simulink model "CLRC_Panda_SP_A"  (R2023a)
settings: Solver=ode3  StartTime=0.0  StopTime=105  FixedStep=Ts  MaxStep=0.005  RelTol=1e-5
model workspace (MAT data in the model file):
  SL_ROS_VariableLengthArrays_MaxSizes.CommonInfo.ArrayTruncateAction = 'EmitWarning'
  SL_ROS_VariableLengthArrays_MaxSizes.MsgTypeMap = containers.Map
  SL_ROS_VariableLengthArrays_MaxSizes.MsgTypeMap.serialization.keys = {'gazebo_msgs/ApplyJointEffortRequest', 'sensor_msgs/JointState'}
  SL_ROS_VariableLengthArrays_MaxSizes.MsgTypeMap.serialization.values{1}.PropertyName = 'JointName'
  SL_ROS_VariableLengthArrays_MaxSizes.MsgTypeMap.serialization.values{1}.DataType = 'uint8'
  SL_ROS_VariableLengthArrays_MaxSizes.MsgTypeMap.serialization.values{1}.MaxLength = 12
  SL_ROS_VariableLengthArrays_MaxSizes.MsgTypeMap.serialization.values{2}(1).PropertyName = 'Effort'
  SL_ROS_VariableLengthArrays_MaxSizes.MsgTypeMap.serialization.values{2}(1).DataType = 'double'
  SL_ROS_VariableLengthArrays_MaxSizes.MsgTypeMap.serialization.values{2}(1).MaxLength = 128
  SL_ROS_VariableLengthArrays_MaxSizes.MsgTypeMap.serialization.values{2}(2).PropertyName = 'Name'
  SL_ROS_VariableLengthArrays_MaxSizes.MsgTypeMap.serialization.values{2}(2).DataType = 'std_msgs/String'
  SL_ROS_VariableLengthArrays_MaxSizes.MsgTypeMap.serialization.values{2}(2).MaxLength = 16
  SL_ROS_VariableLengthArrays_MaxSizes.MsgTypeMap.serialization.values{2}(3).PropertyName = 'Position'
  SL_ROS_VariableLengthArrays_MaxSizes.MsgTypeMap.serialization.values{2}(3).DataType = 'double'
  SL_ROS_VariableLengthArrays_MaxSizes.MsgTypeMap.serialization.values{2}(3).MaxLength = 7
  SL_ROS_VariableLengthArrays_MaxSizes.MsgTypeMap.serialization.values{2}(4).PropertyName = 'Velocity'
  SL_ROS_VariableLengthArrays_MaxSizes.MsgTypeMap.serialization.values{2}(4).DataType = 'double'
  SL_ROS_VariableLengthArrays_MaxSizes.MsgTypeMap.serialization.values{2}(4).MaxLength = 7
  SL_ROS_VariableLengthArrays_MaxSizes.MsgTypeMap.serialization.uniformity = 0
  SL_ROS_VariableLengthArrays_MaxSizes.MsgTypeMap.serialization.keyType = 'char'
  SL_ROS_VariableLengthArrays_MaxSizes.MsgTypeMap.serialization.valueType = 'any'
values from neighbouring files (symbols this model uses):
  B = 4.44*I    [Panda_run.m]
  D = 0.1075*I    [Panda_run.m]
  eKd = 1*inv(K)*B*2*omega_n-inv(K)*D    [Panda_run.m]
  K = 14000*I    [Panda_run.m]
  Kc = diag([20,20,20,20,8,8,5])*0.5    [Panda_run.m]
  Kp = kpdata    [Kp_Compare.m]    (also in Panda_run.m = kp*I)
  Lambda = 10*eye(7)*0.5    [Panda_run.m]
  par = baseparmes()    [Panda_run.m]
  q0 = traj.qd.Data(:,:,1)    [Panda_run.m]
  SD = 0    [Panda_run.m]
  Ts = 0.0005    [Kp_Compare.m]    (also in Panda_run.m)
  vari = SD^2    (= 0)    [Panda_run.m]
undefined symbols (not defined in the file or in its folder): gravityMatrix
libraries: matrix_library x1
settings Model: Creator=STT  LastModifiedBy=stt
settings OptimizationCC: DefaultParameterBehavior=Inlined  EnhancedBackFolding=on  PassReuseOutputArgsAs=Individual arguments  ZeroExternalMemoryAtStartup=off  ZeroInternalMemoryAtStartup=off  MaxStackSize=64  AccelVerboseBuild=on  OptimizeBlockOrder=speed  DifferentSizesBufferReuse=on  OptimizationCustomize=off  EfficientTunableParamExpr=on
settings DebuggingCC: AlgebraicLoopMsg=error  ArtificialAlgebraicLoopMsg=error  ParameterTunabilityLossMsg=error  UnconnectedInputMsg=warning  UnconnectedOutputMsg=warning  UnconnectedLineMsg=warning
settings HardwareCC: ProdHWDeviceType=AMD->x86-64 (Windows64)
settings ModelReferenceCC: EnableRefExpFcnMdlSchedulingChecks=on
settings SFSimCC: MATLABDynamicMemAlloc=off
settings RTWCC: Description=Embedded Coder  SystemTargetFile=ert.tlc  TemplateMakefile=ert_default_tmf  Toolchain=Catkin  DLArmComputeVersion=19.05
settings CodeAppCC: ForceParamTrailComments=on  IgnoreCustomStorageClasses=off  OperatorAnnotations=on  SimulinkDataObjDesc=on  SFDataObjDesc=on  InsertBlockDesc=on
settings ERTTargetCC: SupportContinuousTime=on  SupportVariableSizeSignals=on  ExtMode=on  ExtModeMexArgs='192.168.175.128' 0 17725  ERTCustomFileTemplate=example_file_process.tlc

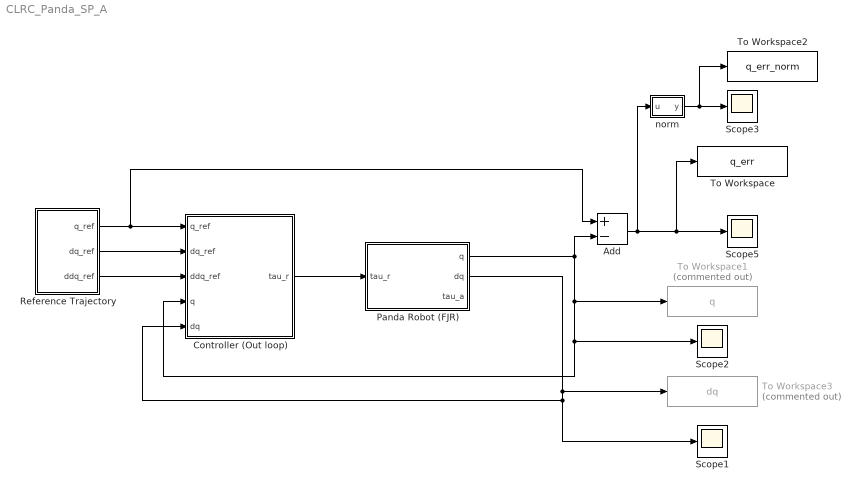
== system CLRC_Panda_SP_A ==
  Add : Sum  Inputs=+-
  Controller (Out loop) : Subsystem
  Panda Robot (FJR) : Subsystem
  Reference Trajectory : Subsystem
  Scope{1..3,5} (4 alike) : Scope
  To Workspace : ToWorkspace  VariableName=q_err  SaveFormat=Timeseries  SampleTime=-1
  To Workspace1 : ToWorkspace  Commented=on  VariableName=q  SaveFormat=Timeseries  SampleTime=-1
  To Workspace2 : ToWorkspace  VariableName=q_err_norm  SaveFormat=Timeseries  SampleTime=-1
  To Workspace3 : ToWorkspace  Commented=on  VariableName=dq  SaveFormat=Timeseries  SampleTime=-1
  norm : MATLAB Function  TreatAsAtomicUnit=on
  wires:
  Reference Trajectory/1(q_ref) -> Add/1, Controller (Out loop)/1(q_ref)
  Reference Trajectory/2(dq_ref) -> Controller (Out loop)/2(dq_ref)
  Reference Trajectory/3(ddq_ref) -> Controller (Out loop)/3(ddq_ref)
  Add/1 -> norm/1(u), Scope5/1, To Workspace/1
  Panda Robot (FJR)/2(dq) -> Scope1/1, Controller (Out loop)/5(dq), To Workspace3/1
  Panda Robot (FJR)/1(q) -> Add/2, Controller (Out loop)/4(q), Scope2/1, To Workspace1/1
  norm/1(y) -> To Workspace2/1, Scope3/1
  Controller (Out loop)/1(tau_r) -> Panda Robot (FJR)/1(tau_r)

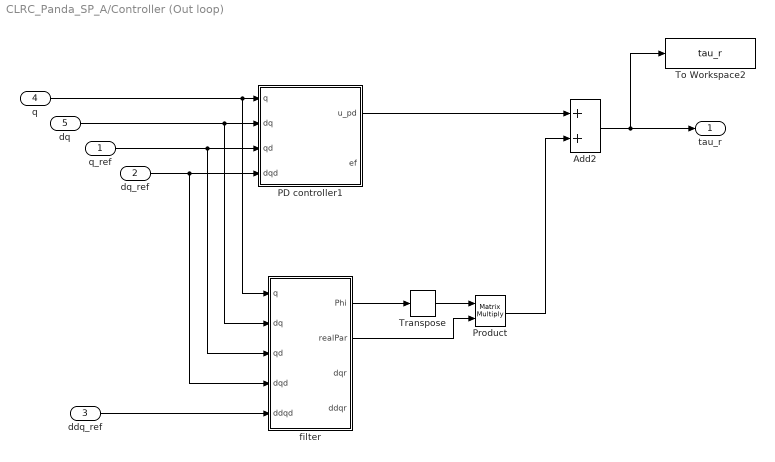
== system CLRC_Panda_SP_A/Controller (Out loop) ==
  q_ref : Inport
  dq_ref : Inport  Port=2
  ddq_ref : Inport  Port=3
  q : Inport  Port=4
  dq : Inport  Port=5
  Add2 : Sum
  PD controller1 : Subsystem
  Product : Product  Multiplication=Matrix(*)
  To Workspace2 : ToWorkspace  VariableName=tau_r  SaveFormat=Timeseries  SampleTime=-1
  Transpose : matrix_library/Transpose
  filter : Subsystem
  tau_r : Outport
  wires:
  q/1 -> PD controller1/1(q), filter/1(q)
  q_ref/1 -> PD controller1/3(qd), filter/3(qd)
  dq_ref/1 -> PD controller1/4(dqd), filter/4(dqd)
  dq/1 -> PD controller1/2(dq), filter/2(dq)
  PD controller1/1(u_pd) -> Add2/1
  Transpose/1 -> Product/1
  Product/1 -> Add2/2
  filter/1(Phi) -> Transpose/1
  filter/2(realPar) -> Product/2
  ddq_ref/1 -> filter/5(ddqd)
  Add2/1 -> tau_r/1, To Workspace2/1

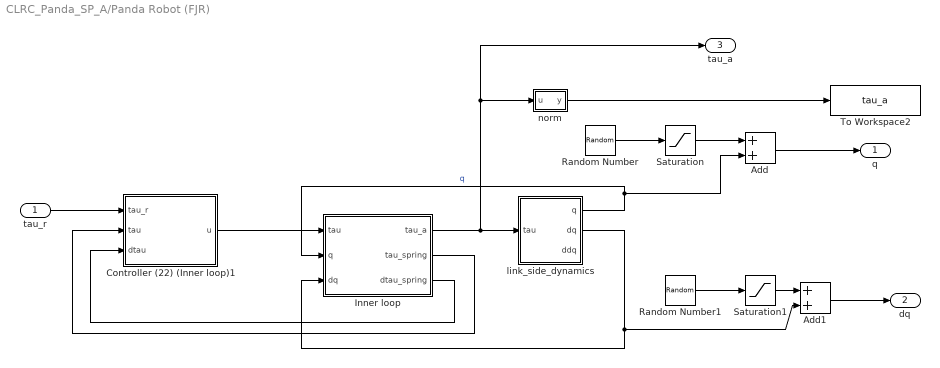
== system CLRC_Panda_SP_A/Panda Robot (FJR) ==
  tau_r : Inport
  Add : Sum
  Add1 : Sum
  Controller (22) (Inner loop)1 : Subsystem
  Inner loop : Subsystem
  Random Number : RandomNumber  Variance=vari  SampleTime=Ts
  Random Number1 : RandomNumber  Variance=vari  SampleTime=Ts
  Saturation : Saturate  UpperLimit=3*SD  LowerLimit=-3*SD
  Saturation1 : Saturate  UpperLimit=3*SD  LowerLimit=-3*SD
  To Workspace2 : ToWorkspace  VariableName=tau_a  SaveFormat=Timeseries  SampleTime=-1
  link_side_dynamics : Subsystem
  norm : MATLAB Function  TreatAsAtomicUnit=on
  q : Outport
  dq : Outport  Port=2
  tau_a : Outport  Port=3
  wires:
  link_side_dynamics/1(q) -> Add/2, Inner loop/2(q)  "q"
  Inner loop/2(tau_spring) -> Controller (22) (Inner loop)1/2(tau)
  Inner loop/3(dtau_spring) -> Controller (22) (Inner loop)1/3(dtau)
  link_side_dynamics/2(dq) -> Inner loop/3(dq), Add1/2
  Controller (22) (Inner loop)1/1(u) -> Inner loop/1(tau)
  norm/1(y) -> To Workspace2/1
  Inner loop/1(tau_a) -> tau_a/1, norm/1(u), link_side_dynamics/1(tau)
  tau_r/1 -> Controller (22) (Inner loop)1/1(tau_r)
  Random Number1/1 -> Saturation1/1
  Saturation/1 -> Add/1
  Random Number/1 -> Saturation/1
  Add/1 -> q/1
  Saturation1/1 -> Add1/1
  Add1/1 -> dq/1

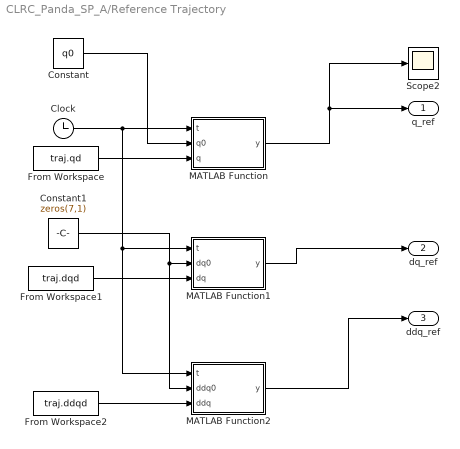
== system CLRC_Panda_SP_A/Reference Trajectory ==
  Clock : Clock
  Constant : Constant  Value=q0
  Constant1 : Constant  Value=zeros(7,1)
  From Workspace : FromWorkspace  VariableName=traj.qd
  From Workspace1 : FromWorkspace  VariableName=traj.dqd
  From Workspace2 : FromWorkspace  VariableName=traj.ddqd
  MATLAB Function : MATLAB Function  TreatAsAtomicUnit=on
  MATLAB Function1 : MATLAB Function  TreatAsAtomicUnit=on
  MATLAB Function2 : MATLAB Function  TreatAsAtomicUnit=on
  Scope2 : Scope
  q_ref : Outport
  dq_ref : Outport  Port=2
  ddq_ref : Outport  Port=3
  wires:
  MATLAB Function/1(y) -> Scope2/1, q_ref/1
  MATLAB Function1/1(y) -> dq_ref/1
  MATLAB Function2/1(y) -> ddq_ref/1
  Clock/1 -> MATLAB Function2/1(t), MATLAB Function1/1(t), MATLAB Function/1(t)
  From Workspace/1 -> MATLAB Function/3(q)
  Constant/1 -> MATLAB Function/2(q0)
  From Workspace1/1 -> MATLAB Function1/3(dq)
  From Workspace2/1 -> MATLAB Function2/3(ddq)
  Constant1/1 -> MATLAB Function2/2(ddq0), MATLAB Function1/2(dq0)

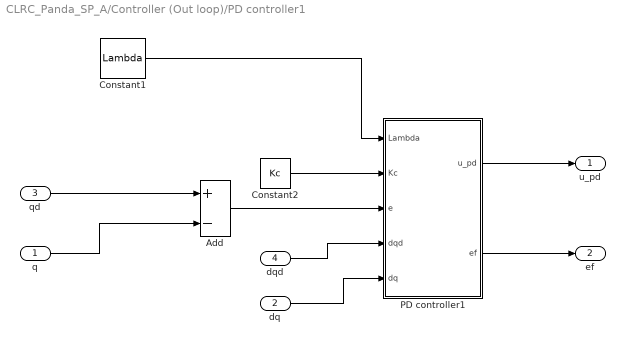
== system CLRC_Panda_SP_A/Controller (Out loop)/PD controller1 ==
  q : Inport
  dq : Inport  Port=2
  qd : Inport  Port=3
  dqd : Inport  Port=4
  Add : Sum  Inputs=+-
  Constant1 : Constant  Value=Lambda
  Constant2 : Constant  Value=Kc
  PD controller1 : MATLAB Function  TreatAsAtomicUnit=on
  u_pd : Outport
  ef : Outport  Port=2
  wires:
  PD controller1/1(u_pd) -> u_pd/1
  Add/1 -> PD controller1/3(e)
  Constant1/1 -> PD controller1/1(Lambda)
  Constant2/1 -> PD controller1/2(Kc)
  PD controller1/2(ef) -> ef/1
  q/1 -> Add/2
  qd/1 -> Add/1
  dq/1 -> PD controller1/5(dq)
  dqd/1 -> PD controller1/4(dqd)

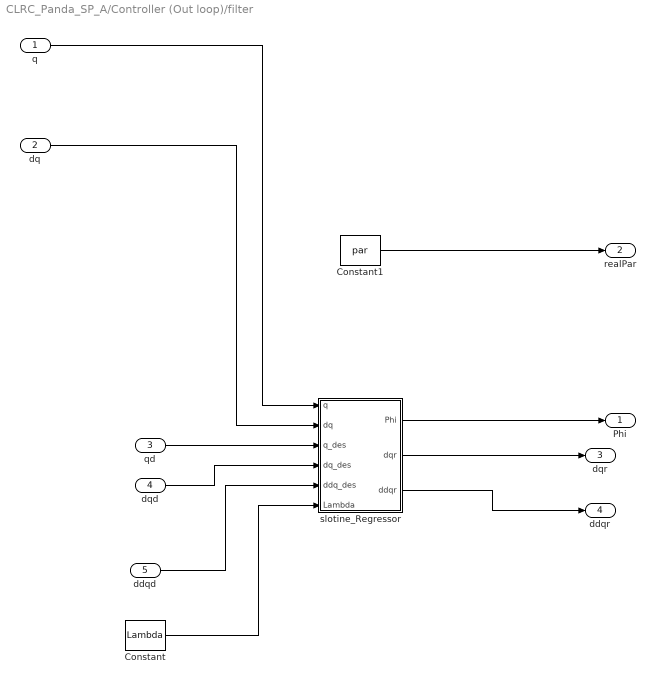
== system CLRC_Panda_SP_A/Controller (Out loop)/filter ==
  q : Inport
  dq : Inport  Port=2
  qd : Inport  Port=3
  dqd : Inport  Port=4
  ddqd : Inport  Port=5
  Constant : Constant  Value=Lambda
  Constant1 : Constant  Value=par
  slotine_Regressor : MATLAB Function  TreatAsAtomicUnit=on
  Phi : Outport
  realPar : Outport  Port=2
  dqr : Outport  Port=3
  ddqr : Outport  Port=4
  wires:
  qd/1 -> slotine_Regressor/3(q_des)
  dqd/1 -> slotine_Regressor/4(dq_des)
  ddqd/1 -> slotine_Regressor/5(ddq_des)
  Constant/1 -> slotine_Regressor/6(Lambda)
  q/1 -> slotine_Regressor/1(q)
  dq/1 -> slotine_Regressor/2(dq)
  Constant1/1 -> realPar/1
  slotine_Regressor/1(Phi) -> Phi/1
  slotine_Regressor/2(dqr) -> dqr/1
  slotine_Regressor/3(ddqr) -> ddqr/1

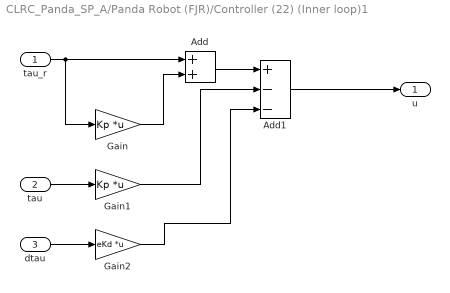
== system CLRC_Panda_SP_A/Panda Robot (FJR)/Controller (22) (Inner loop)1 ==
  tau_r : Inport
  tau : Inport  Port=2
  dtau : Inport  Port=3
  Add : Sum
  Add1 : Sum  Inputs=+--
  Gain : Gain  Gain=Kp  Multiplication=Matrix(K*u)
  Gain1 : Gain  Gain=Kp  Multiplication=Matrix(K*u)
  Gain2 : Gain  Gain=eKd  Multiplication=Matrix(K*u)
  u : Outport
  wires:
  tau/1 -> Gain1/1
  Add/1 -> Add1/1
  Add1/1 -> u/1
  dtau/1 -> Gain2/1
  Gain1/1 -> Add1/2
  tau_r/1 -> Add/1, Gain/1
  Gain/1 -> Add/2
  Gain2/1 -> Add1/3

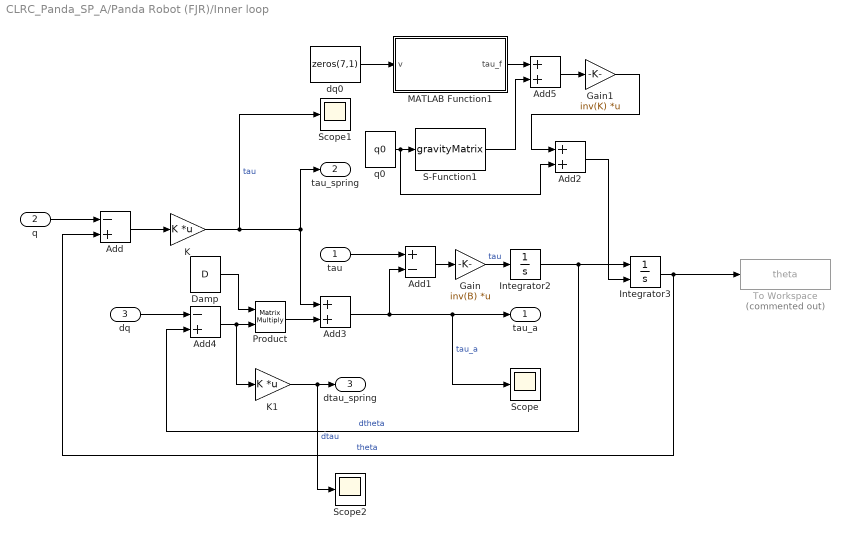
== system CLRC_Panda_SP_A/Panda Robot (FJR)/Inner loop ==
  tau : Inport
  q : Inport  Port=2
  dq : Inport  Port=3
  Add : Sum  Inputs=-+
  Add1 : Sum  Inputs=+-
  Add2 : Sum
  Add3 : Sum
  Add4 : Sum  Inputs=-+
  Add5 : Sum
  Damp : Constant  Value=D
  Gain : Gain  Gain=inv(B)  Multiplication=Matrix(K*u)
  Gain1 : Gain  Gain=inv(K)  Multiplication=Matrix(K*u)
  Integrator2 : Integrator
  Integrator3 : Integrator  InitialConditionSource=external  InitialCondition=q0+K\gravityMatrix(q0)
  K : Gain  Gain=K  Multiplication=Matrix(K*u)
  K1 : Gain  Gain=K  Multiplication=Matrix(K*u)
  MATLAB Function1 : MATLAB Function  TreatAsAtomicUnit=on
  Product : Product  Multiplication=Matrix(*)
  S-Function1 : S-Function  FunctionName=gravityMatrix  SFunctionDeploymentMode=off  EnableBusSupport=off
  Scope : Scope
  Scope1 : Scope
  Scope2 : Scope
  To Workspace : ToWorkspace  Commented=on  VariableName=theta  SaveFormat=Timeseries  SampleTime=-1
  dq0 : Constant  Value=zeros(7,1)
  q0 : Constant  Value=q0
  tau_a : Outport
  tau_spring : Outport  Port=2
  dtau_spring : Outport  Port=3
  wires:
  q/1 -> Add/1
  Add/1 -> K/1
  K/1 -> Scope1/1, tau_spring/1, Add3/1  "tau"
  Product/1 -> Add3/2
  Add1/1 -> Gain/1
  Integrator2/1 -> Integrator3/1, Add4/2  "dtheta"
  Integrator3/1 -> Add/2, To Workspace/1  "theta"
  Add3/1 -> Scope/1, tau_a/1, Add1/2  "tau_a"
  dq/1 -> Add4/1
  Add4/1 -> K1/1, Product/2
  Damp/1 -> Product/1
  K1/1 -> Scope2/1, dtau_spring/1  "dtau"
  tau/1 -> Add1/1
  q0/1 -> Add2/2, S-Function1/1
  Gain1/1 -> Add2/1
  Add2/1 -> Integrator3/2
  dq0/1 -> MATLAB Function1/1(v)
  MATLAB Function1/1(tau_f) -> Add5/1
  Add5/1 -> Gain1/1
  S-Function1/1 -> Add5/2
  Gain/1 -> Integrator2/1  "tau"

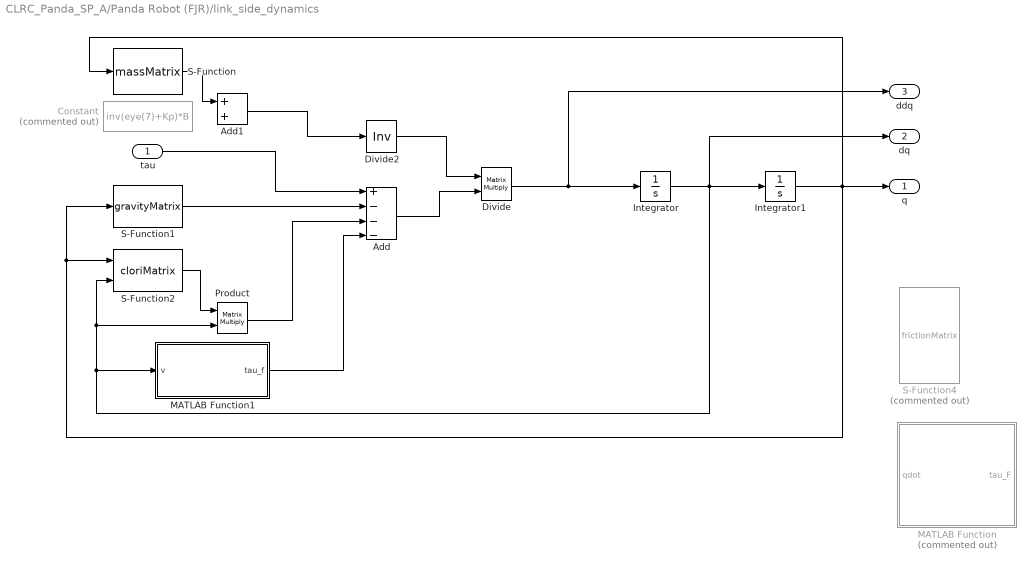
== system CLRC_Panda_SP_A/Panda Robot (FJR)/link_side_dynamics ==
  tau : Inport
  Add : Sum  Inputs=+---
  Add1 : Sum
  Constant : Constant  Commented=on  Value=inv(eye(7)+Kp)*B
  Divide : Product  Inputs=**  Multiplication=Matrix(*)
  Divide2 : Product  Inputs=/  Multiplication=Matrix(*)
  Integrator : Integrator
  Integrator1 : Integrator  InitialCondition=q0
  MATLAB Function : MATLAB Function  Commented=on  TreatAsAtomicUnit=on
  MATLAB Function1 : MATLAB Function  TreatAsAtomicUnit=on
  Product : Product  Multiplication=Matrix(*)
  S-Function : S-Function  FunctionName=massMatrix  SFunctionDeploymentMode=off  EnableBusSupport=off
  S-Function1 : S-Function  FunctionName=gravityMatrix  SFunctionDeploymentMode=off  EnableBusSupport=off
  S-Function2 : S-Function  FunctionName=cloriMatrix  SFunctionDeploymentMode=off  EnableBusSupport=off
  S-Function4 : S-Function  Commented=on  FunctionName=frictionMatrix  SFunctionDeploymentMode=off  EnableBusSupport=off
  q : Outport
  dq : Outport  Port=2
  ddq : Outport  Port=3
  wires:
  Integrator1/1 -> S-Function/1, q/1, S-Function1/1, S-Function2/1
  S-Function1/1 -> Add/2
  S-Function2/1 -> Product/1
  Divide/1 -> ddq/1, Integrator/1
  Integrator/1 -> Integrator1/1, MATLAB Function1/1(v), Product/2, S-Function2/2, dq/1
  Product/1 -> Add/3
  tau/1 -> Add/1
  Add/1 -> Divide/2
  Divide2/1 -> Divide/1
  MATLAB Function1/1(tau_f) -> Add/4
  S-Function/1 -> Add1/1
  Add1/1 -> Divide2/1

== matlab function CLRC_Panda_SP_A/Controller (Out loop)/filter/slotine_Regressor ==
  data: q input; Phi output; dq input; q_des input; dq_des input; ddq_des input; Lambda input; dqr output; ddqr output
function [Phi,dqr,ddqr]= fcn(q,dq,q_des,dq_des,ddq_des,Lambda)
e1=q-q_des;
de1=dq-dq_des;
dqr=dq_des-Lambda*e1;
ddqr=ddq_des-Lambda*de1;

Phi=Base_Slotine_Panda(q,dq,dqr,ddqr);

== matlab function CLRC_Panda_SP_A/Panda Robot (FJR)/norm ==
  data: u input; y output
function y= fcn(u)

y = norm(u);

== matlab function CLRC_Panda_SP_A/norm ==
  data: u input; y output
function y= fcn(u)

y = norm(u);

== matlab function CLRC_Panda_SP_A/Reference Trajectory/MATLAB Function ==
  data: t input; y output; q0 input; q input
function y = fcn(t,q0,q)
if t<=25
    y=q;
elseif t>=75 && t<=100
    y=q;
else
    y=q0;
end

== matlab function CLRC_Panda_SP_A/Reference Trajectory/MATLAB Function1 ==
  data: t input; y output; dq0 input; dq input
function y = fcn(t,dq0,dq)
if t<=25
    y=dq;
elseif t>=75 && t<=100
    y=dq;
else
    y=dq0;
end

== matlab function CLRC_Panda_SP_A/Reference Trajectory/MATLAB Function2 ==
  data: t input; y output; ddq0 input; ddq input
function y = fcn(t,ddq0,ddq)
if t<=25
    y=ddq;
elseif t>=75 && t<=100
    y=ddq;
else
    y=ddq0;
end

== matlab function CLRC_Panda_SP_A/Controller (Out loop)/PD controller1/PD controller1 ==
  data: Lambda input; Kc input; e input; dqd input; u_pd output; dq input; ef output
function [u_pd,ef]= fcn(Lambda,Kc,e,dqd,dq)

dqr=dqd+Lambda*e;

ef=dqr-dq;

u_pd = Kc*ef;

== matlab function CLRC_Panda_SP_A/Panda Robot (FJR)/link_side_dynamics/MATLAB Function ==
  data: qdot input; tau_F output
% author: Claudio Gaz, Marco Cognetti, Alexander Oliva
% date: September 3, 2019
% 
% -------------------------------------------------
% Panda Dynamic Model v. 1.0
% -------------------------------------------------
% C. Gaz, M. Cognetti, A. Oliva, P. Robuffo Giordano, A. De Luca, 'Dynamic
% Identification of the Franka Emika Panda Robot With Retrieval of Feasible
% Parameters Using Penalty-Based Optimization'. IEEE RA-L, 2019.
%
% the following code has been tested on Matlab 2018b

% get_FrictionTorque returns the numerical joint friction torque vector 
% tau_f(qdot), given the current joint velocities

function tau_F = get_FrictionTorque(qdot)

    fp = [...
        0.54615,0.87224,0.64068,1.2794,0.83904,0.30301,0.56489;...
        0,0,0,0,0,0,0;...
        0.039533,0.025882,-0.04607,0.036194,0.026226,-0.021047,0.0035526;...
        5.1181,9.0657,10.136,5.5903,8.3469,17.133,10.336];

    A = fp(1,:);
    k = fp(2,:);
    qdotsign = fp(3,:);
    alpha= fp(4,:);
    
    num_of_joints = length(qdot);
    tau_F = zeros(num_of_joints,1);
    
    for i=1:num_of_joints
        tau_F(i) = -A(i)/(1+exp(-alpha(i)*qdotsign(i))) + A(i)/(1+exp(-alpha(i)*(qdot(i)+qdotsign(i))));
    end

== matlab function CLRC_Panda_SP_A/Panda Robot (FJR)/link_side_dynamics/MATLAB Function1 ==
  data: v input; tau_f output
function tau_f = signFriction(v)
 f_v =[0.0665, 0.1987, 0.0399, 0.2257,  0.1023, -0.0132, 0.0638]';
 f_c =[0.245, 0.1523, 0.1827, 0.3591, 0.2669, 0.1658, 0.2109 ]';
 f_o =[-0.1073,-0.1566,-0.0686,-0.2522,0.0045,0.0910,-0.0127]';
 tau_f = f_v.*v+f_c.*tanh(300*v)+f_o;

== matlab function CLRC_Panda_SP_A/Panda Robot (FJR)/Inner loop/MATLAB Function1 ==
  data: v input; tau_f output
function tau_f = signFriction(v)
 f_v =[0.0665, 0.1987, 0.0399, 0.2257,  0.1023, -0.0132, 0.0638]';
 f_c =[0.245, 0.1523, 0.1827, 0.3591, 0.2669, 0.1658, 0.2109 ]';
 f_o =[-0.1073,-0.1566,-0.0686,-0.2522,0.0045,0.0910,-0.0127]';
 tau_f = f_v.*v+f_c.*tanh(300*v)+f_o;
